simulink model "iap_device_boot_demo"  (Simulink 7.3)
settings: Solver=FixedStepDiscrete  SolverMode=SingleTasking  StartTime=0.0  StopTime=10.0  RelTol=1e-3
PreLoadFcn:
  | waijung.modelPreload; % Required for working with Waijung Blockset. Do not remove.
undefined symbols (not defined in the file): HSEOSC, Link, LQFP176, ST, STM32F417IG
libraries: simulink x22, stm32f4_flash_lib x12, stm32f4_canbus_lib x4, stm32f4_reset_lib x3, stm32f4_io_lib x3, stm32f4_boot_lib x2, stm32f4_crc_lib x2, stm32f4_device_config_lib x1
CloseFcn:
  | waijung.modelClose; % Required for working with Waijung Blockset. Do not remove.
settings Model: Creator=Krisada  LastModifiedBy=Krisada
settings OptimizationCC: OptimizeModelRefInitCode=on  LifeSpan=1
settings HardwareCC: ProdEndianess=LittleEndian  ProdHWDeviceType=ARM Compatible->Cortex - M4  TargetEndianess=LittleEndian  TargetHWDeviceType=ARM Compatible->Cortex - M4
settings RTWCC: SystemTargetFile=stm32f4.tlc  GenerateMakefile=off  TemplateMakefile=ert_default_tmf  Description=STM32F4 Target  ProcessScript=stm32f4_make_rtw_hook
settings CodeAppCC: IgnoreCustomStorageClasses=off
settings STFCustomTargetCC: ModelReferenceCompliant=off  CombineOutputUpdateFcns=on  ERTCustomFileBanners=on  SupportContinuousTime=off  SupportNonInlinedSFcns=off  SystemTargetFile=stm32f4.tlc
settings ERTTargetCC: MultiwordLength=2048  ModelReferenceCompliant=off  ParMdlRefBuildCompliant=off  CompOptLevelCompliant=off  ERTFirstTimeCompliant=off  ModelStepFunctionPrototypeControlCompliant=off  CPPClassGenCompliant=off  ExtModeMexFile=noextcomm  InlinedParameterPlacement=NonHierarchical  ERTSrcFileBannerTemplate=stm32f4_code_template.cgt  ERTHdrFileBannerTemplate=stm32f4_code_template.cgt  ERTDataSrcFileTemplate=stm32f4_code_template.cgt  ERTDataHdrFileTemplate=stm32f4_code_template.cgt  ERTCustomFileTemplate=stm32f4_file_process.tlc

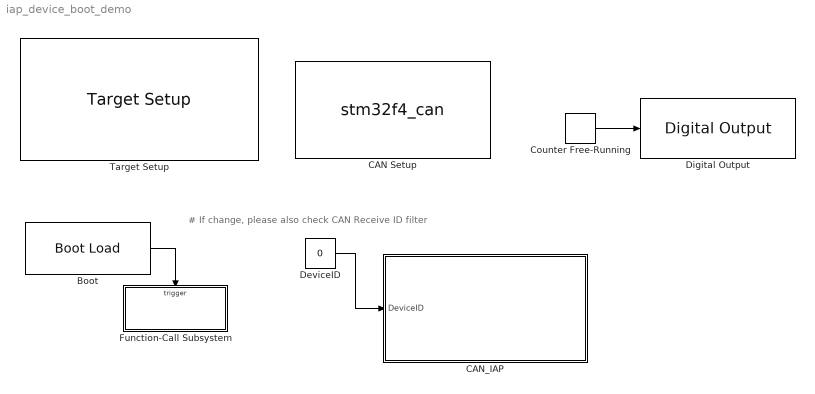
== system iap_device_boot_demo ==
  note: # If change,
      | please also check CAN Receive ID filter
  Boot : stm32f4_boot_lib/Boot Load  conf=Boot  flashorigin=0x8000000  flashlength=0x100000  enableisr=on  usersector=Sector 9: 0x080A0000 - 0x080BFFFF  sampletime=-1  sampletimestr=0.001  blockid=Boot  inputarray=[]  inputlabelarray={}  outputarray=[7]  outputlabelarray={'Call ISR'}  compat=0  confstr="[\"080A0000\",\"9\"]"
  CAN Setup : S-Function  FunctionName=stm32f4_can  Parameters=conf,canmodule,0,inputarray,outputarray,'','',confstr,sampletime,sampletimestr,blockid  EnableBusSupport=off  mask(stm32f4_can){conf=Setup, canmodule=1, advance=off, bitrate_select=125000, sjw=1tq, bs1=14tq, bs2=6tq, timingconf=Prescaler, brp=16, bitrate=125000, tq=3.8095e-007, remaptxpin=B9, remaprxpin=B8, sampletime=inf, sampletimestr=0.001, blockid=CANSetup, inputarray=[], inputlabelarray={}, outputarray=[], outputlabelarray={}, compat=0, confstr=["125000","16","B","9","B","8","1tq","14tq","6tq","ENABLE"], presc=16, txportstr=B, txpinstr=9, rxportstr=B, rxpinstr=8, lastmodule=1}
      mask prompts: conf "Configuration"; canmodule "CAN Module"; advance "Advance configuration"; bitrate_select "Baud rate (bps)"; sjw "Resync Jump Width (SJW)"; bs1 "Bit segment 1 (BS1) + PROP_SEG"; bs2 "Bit segment 2 (BS2)"; timingconf "Adjust"; brp "Baud rate prescaler (BRP)"; bitrate "Baud rate (bps)"; tq "Time Quantum (Second), tq"; remaptxpin "CAN Tx pin"; remaprxpin "CAN Rx pin"; sampletime "Sample time (sec)"; sampletimestr "Compiled sample time (sec) in string"; inputarray "Input port"; inputlabelarray "Input port label"; outputarray "Output port"; outputlabelarray "Output port label"; compat "Compatibility (Reserved for future use)"; confstr "Configuration String"; presc "Prescale"; txportstr "Tx port string"; txpinstr "Tx pin string"; rxportstr "Rx port string"; rxpinstr "Rx pin string"; lastmodule "Last module selected"
      mask help: This block setups CAN Module.
      mask init:
      | stm32f4_can_callback('init');
      mask Help: web(fullfile(waijungdocroot,'stm32f4_can_setup.htm'), '-browser')
      mask StyleString: popup(Setup),popup(1|2),checkbox,popup(125000|250000|500000|1000000),popup(1tq|2tq|3tq|4tq),popup(1tq|2tq|3tq|4tq|5tq|6tq|7tq|8tq|9tq|10tq|11tq|12tq|13tq|14tq|15tq|16tq),popup(1tq|2tq|3tq|4tq|5tq|6tq|7tq|8tq),popup(Prescaler|Baudrate),edit,edit,edit,popup(Not used|A12|B9|D1|H13),popup(Not used|A11|B8|D0|I9),edit,edit,edit,edit,edit,edit,edit,edit,edit,edit,edit,edit,edit,edit,edit
      mask CallbackString: |stm32f4_can_callback('canmodule');|stm32f4_can_callback('advance');|stm32f4_can_callback('bitrate_select');||stm32f4_can_callback('timingconf');|stm32f4_can_callback('timingconf');|stm32f4_can_callback('timingconf');|stm32f4_can_callback('timingconf');|stm32f4_can_callback('timingconf');||stm32f4_can_callback('remaptxpin');|stm32f4_can_callback('remaprxpin');|stm32f4_can_callback('sampletime');|stm32f4_can_callback('sampletimestr');|stm32f4_can_callback('blockid');||||||||||||
      mask Display: text(0.5, 0.5, 'CAN1_Setup\nSpeed (bps): 125000\nTx/Rx pin: B9/B8','ver','middle','hor','center');
  CAN_IAP : Subsystem  TreatAsAtomicUnit=on
  Counter Free-Running : simulink/Sources/Counter Free-Running  SystemSampleTime=-1  NumBits=16  tsamp=0.5
  DeviceID : Constant  Value=0  OutDataTypeMode=uint32  OutDataType=fixdt(1, 16)  OutScaling=2^0  OutDataTypeStr=uint32  SampleTime=0.001
  Digital Output : stm32f4_io_lib/Digital Output  use_bitband=on  port=D  speed=100  porttype=Push Pull  porttypestr=PP  use_pin0=off  use_pin1=off  use_pin2=off  use_pin3=off  use_pin4=off  use_pin5=off  use_pin6=off  use_pin7=off  use_pin8=off  use_pin9=off  use_pin10=off  use_pin11=off  use_pin12=off  use_pin13=off  use_pin14=off  use_pin15=on  pinstr=GPIO_Pin_15  usedpinarray="[0  0  0  0  0  0  0  0  0  0  0  0  0  0  0  1]"  bitbandingstr="#define DigitalOutput_D15 Peripheral_BB(GPIOD->ODR, 15)  /* Output pin */"  sampletime=-1  sampletimestr=0.5  blockid=DigitalOutput  enablecustomportlabel=off  globalinit=off  cinputportlabel=In1, In2  coutputportlabel=0
  Function-Call Subsystem : Subsystem  TreatAsAtomicUnit=on
  Target Setup : stm32f4_device_config_lib/Target Setup  Priority=100  compiler=GNU ARM  previous_compiler=GNU ARM  mcu=STM32F417IG (LQFP176)  mcustr=STM32F417IG  clockconfig=HSEOSC-8MHz  system_stm32f4xx_c_path=F:\trunk\targets\stm32f4_target\stm32f4\utils\system_stm32f4xx_default\STM32F40_41xxx\hseosc8mhz  showmemoryconfiguration=off  stacksize=0x2000  heapsize=0x2000  enableautocompiledownload=on  fullchiperase=on  programmerinterface=ST-Link  editctrlstr=on  compilercontrolstr=$(patsubst %, -I%, .) -mcpu=cortex-m4 -mthumb -mthumb-interwork -mfloat-abi=hard -mfpu=fpv4-sp-d16 -ffast-math -Wall -Wextra -Ofast  assemblercontrolstr=$(patsubst %, -I%, .) -mcpu=cortex-m4 -mthumb -mthumb-interwork -mfloat-abi=hard -mfpu=fpv4-sp-d16 -ffast-math -Wall -Wextra -Ofast -Wa,-amhls=$(<:.s=.lst) -D__STACK_SIZE=$(STACK_SIZE) -D__HEAP_SIZE=$(HEAP_SIZE)  linkercontrolstr=-T$(LD_SCRIPT) -g -Wl,-Map=$(MAP),--cref,--no-warn-mismatch -mcpu=cortex-m4 -mthumb -mthumb-interwork -mfloat-abi=hard -mfpu=fpv4-sp-d16 -specs=nosys.specs  runafterdownload=on  execprofile=None  profileruart=3  profilerbaud=500000  profilertxpin=D8  profilerinitstr=0.001,168000000,168000,500000,0  manualsetsampletime=off  sampletime=0.001  blockid=TargetSetup  systickreloadvalue=168000  hseval=8000000  lastprofileruart=3  hclk=168000000  flashorigin=0x8000000  flashlength=1024k  ramorigin=0x20000000  ramlength=128k  useextram=off
  wires:
  Boot/1 -> Function-Call Subsystem/Trigger
  DeviceID/1 -> CAN_IAP/1(DeviceID)
  Counter Free-Running/1 -> Digital Output/1

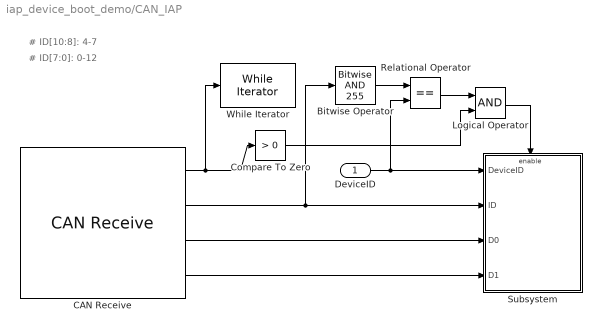
== system iap_device_boot_demo/CAN_IAP ==
  note: # ID[7:0]: 0-12
  note: # ID[10:8]: 4-7
  DeviceID : Inport  OutDataType=fixdt(1, 16)  OutScaling=2^0
  Bitwise Operator : simulink/Logic and Bit Operations/Bitwise Operator  logicop=AND  UseBitMask=on  BitMask=255  BitMaskRealWorld=Stored Integer
  CAN Receive : stm32f4_canbus_lib/CAN Receive  conf=Rx  canmodule=1  idtype=Standard  filtertype=Mask  id=hex2dec('400')  idmask=hex2dec('4F0')  enableisr=off  usedlc=off  datatype=uint32  data0type=uint32  data1type=uint32  data2type=Not used  data3type=Not used  data4type=Not used  data5type=Not used  data6type=Not used  data7type=Not used  buffersize=32  sampletime=-1  sampletimestr=-1  blockid=CAN_IAPCANReceive  inputarray=[]  inputlabelarray={}  outputarray=[ 5, 7, 7, 7]  outputlabelarray={ 'Msg Pending','ID', 'D0 (uint32)', 'D1 (uint32)' }  compat=0  confstr="[\"Standard\",\"Mask\",\"1024\",\"1264\",\"off\",\"uint32\",\"uint32\",\"Not used\",\"Not used\",\"Not used\",\"Not used\",\"Not used\",\"Not used\",\"32\",\"8000\",\"0\",\"9E00\",\"4\"]"
  Compare To Zero : simulink/Logic and Bit Operations/Compare To Zero  SystemSampleTime=-1  relop=>  LogicOutDataTypeMode=uint8  ZeroCross=off
  Logical Operator : Logic  AllPortsSameDT=off  OutDataTypeMode=boolean  LogicDataType=fixdt(0, 8)  OutDataTypeStr=boolean
  Relational Operator : RelationalOperator  Operator===  LogicOutDataTypeMode=boolean  LogicDataType=fixdt(0, 8)  OutDataTypeStr=boolean
  Subsystem : Subsystem
  While Iterator : WhileIterator  WhileBlockType=do-while
  wires:
  CAN Receive/1 -> Compare To Zero/1, While Iterator/1
  CAN Receive/4 -> Subsystem/4(D1)
  CAN Receive/2 -> Subsystem/2(ID), Bitwise Operator/1
  CAN Receive/3 -> Subsystem/3(D0)
  Relational Operator/1 -> Logical Operator/1
  Compare To Zero/1 -> Logical Operator/2
  Logical Operator/1 -> Subsystem/Enable
  Bitwise Operator/1 -> Relational Operator/1
  DeviceID/1 -> Subsystem/1(DeviceID), Relational Operator/2

== system iap_device_boot_demo/Function-Call Subsystem ==
  note: # 1. Stay in boot if PA0 pressed during Startup
  note: 2. Otherwise, check flash healthy
  function : TriggerPort  TriggerType=function-call
  Check Boot Pin : Subsystem  TreatAsAtomicUnit=on
  Check Flash : Subsystem
  Constant : Constant  OutDataType=fixdt(1, 16)  OutScaling=2^0
  wires:
  Constant/1 -> Check Boot Pin/Enable
  Check Boot Pin/1(Out1) -> Check Flash/Enable

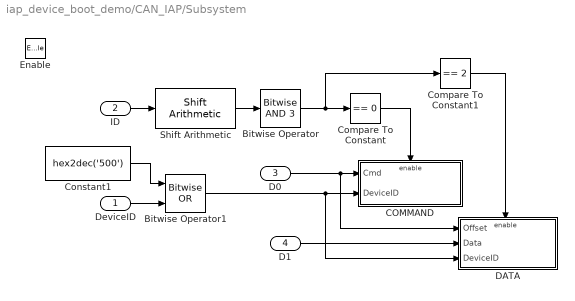
== system iap_device_boot_demo/CAN_IAP/Subsystem ==
  DeviceID : Inport
  ID : Inport  Port=2
  D0 : Inport  Port=3
  D1 : Inport  Port=4
  Enable : EnablePort
  Bitwise Operator : simulink/Logic and Bit Operations/Bitwise Operator  logicop=AND  UseBitMask=on  BitMask=3  BitMaskRealWorld=Stored Integer
  Bitwise Operator1 : simulink/Logic and Bit Operations/Bitwise Operator  logicop=OR  UseBitMask=off  NumInputPorts=2  BitMask=bin2dec('11011001')  BitMaskRealWorld=Stored Integer
  COMMAND : Subsystem  TreatAsAtomicUnit=on
  Compare To Constant : simulink/Logic and Bit Operations/Compare To Constant  SystemSampleTime=-1  relop===  const=0  LogicOutDataTypeMode=uint8  ZeroCross=off
  Compare To Constant1 : simulink/Logic and Bit Operations/Compare To Constant  SystemSampleTime=-1  relop===  const=2  LogicOutDataTypeMode=uint8  ZeroCross=off
  Constant1 : Constant  Value=hex2dec('500')  OutDataTypeMode=uint32  OutDataType=fixdt(1, 16)  OutScaling=2^0  OutDataTypeStr=uint32
  DATA : Subsystem  TreatAsAtomicUnit=on
  Shift Arithmetic : simulink/Logic and Bit Operations/Shift Arithmetic  SystemSampleTime=-1  nBitShiftRight=8  nBinPtShiftRight=0
  wires:
  Shift Arithmetic/1 -> Bitwise Operator/1
  Bitwise Operator/1 -> Compare To Constant1/1, Compare To Constant/1
  Compare To Constant/1 -> COMMAND/Enable
  D0/1 -> COMMAND/1(Cmd), DATA/1(Offset)
  Compare To Constant1/1 -> DATA/Enable
  ID/1 -> Shift Arithmetic/1
  D1/1 -> DATA/2(Data)
  Constant1/1 -> Bitwise Operator1/1
  DeviceID/1 -> Bitwise Operator1/2
  Bitwise Operator1/1 -> COMMAND/2(DeviceID), DATA/3(DeviceID)

== system iap_device_boot_demo/Function-Call Subsystem/Check Boot Pin ==
  Enable : EnablePort
  Digital Input : stm32f4_io_lib/Digital Input  port=A  speed=100  porttype=None  porttypestr=NOPULL  use_pin0=on  use_pin1=off  use_pin2=off  use_pin3=off  use_pin4=off  use_pin5=off  use_pin6=off  use_pin7=off  use_pin8=off  use_pin9=off  use_pin10=off  use_pin11=off  use_pin12=off  use_pin13=off  use_pin14=off  use_pin15=off  pinstr=GPIO_Pin_0  usedpinarray="[1  0  0  0  0  0  0  0  0  0  0  0  0  0  0  0]"  bitbandingstr="#define FunctionCallSubsystemCheckBootPinDigitalInput_A0 Peripheral_BB(GPIOA->IDR, 0)  /* Output pin */"  sampletime=inf  sampletimestr=-1  blockid=FunctionCallSubsystemCheckBootPinDigitalInput  enablecustomportlabel=off  glabalinit=off  cinputportlabel=In1, In2  coutputportlabel=Out1, Out2
  Logical Operator : Logic  Operator=NOT  AllPortsSameDT=off  OutDataTypeMode=boolean  LogicDataType=fixdt(0, 8)  OutDataTypeStr=boolean
  Out1 : Outport  OutDataType=fixdt(1, 16)  OutScaling=2^0
  wires:
  Digital Input/1 -> Logical Operator/1
  Logical Operator/1 -> Out1/1

== system iap_device_boot_demo/Function-Call Subsystem/Check Flash ==
  note: #  Check if firmwar has valid stack address,
      | reduce proces to check CRC32 when firmware invalid
  note: ### Sector C location: Sector_6
  Enable : EnablePort
  Check Sector B : Subsystem  TreatAsAtomicUnit=on
  Check Sector C : Subsystem
  Logical Operator : Logic  Operator=NOT  AllPortsSameDT=off  OutDataTypeMode=boolean  LogicDataType=fixdt(0, 8)  OutDataTypeStr=boolean
  Upgrade Firmware : Subsystem  TreatAsAtomicUnit=on
  wires:
  Check Sector C/1(Sector Valid) -> Upgrade Firmware/Enable, Logical Operator/1
  Logical Operator/1 -> Check Sector B/Enable

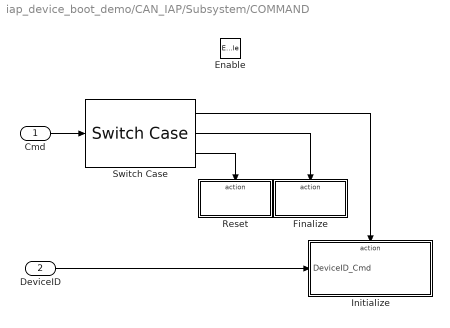
== system iap_device_boot_demo/CAN_IAP/Subsystem/COMMAND ==
  Cmd : Inport  OutDataType=fixdt(1, 16)  OutScaling=2^0
  DeviceID : Inport  Port=2  OutDataType=fixdt(1, 16)  OutScaling=2^0
  Enable : EnablePort
  Finalize : Subsystem  TreatAsAtomicUnit=on
  Initialize : Subsystem  TreatAsAtomicUnit=on
  Reset : Subsystem  TreatAsAtomicUnit=on
  Switch Case : SwitchCase  CaseConditions={0,1,2}  CaseShowDefault=off
  wires:
  Cmd/1 -> Switch Case/1
  Switch Case/1 -> Initialize/Action
  Switch Case/2 -> Finalize/Action
  Switch Case/3 -> Reset/Action
  DeviceID/1 -> Initialize/1(DeviceID_Cmd)

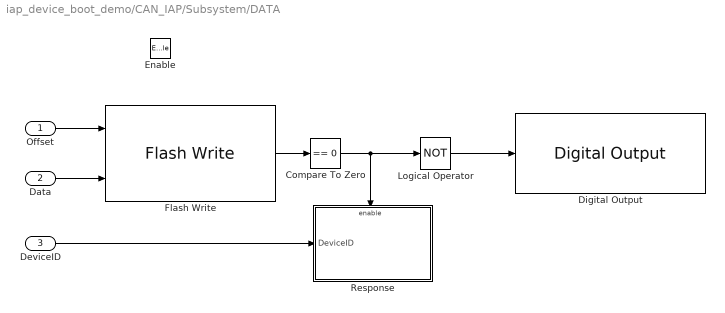
== system iap_device_boot_demo/CAN_IAP/Subsystem/DATA ==
  Offset : Inport  OutDataType=fixdt(1, 16)  OutScaling=2^0
  Data : Inport  Port=2  OutDataType=fixdt(1, 16)  OutScaling=2^0
  DeviceID : Inport  Port=3  OutDataType=fixdt(1, 16)  OutScaling=2^0
  Enable : EnablePort
  Compare To Zero : simulink/Logic and Bit Operations/Compare To Zero  SystemSampleTime=-1  relop===  LogicOutDataTypeMode=uint8  ZeroCross=off
  Digital Output : stm32f4_io_lib/Digital Output  use_bitband=on  port=D  speed=100  porttype=Push Pull  porttypestr=PP  use_pin0=off  use_pin1=off  use_pin2=off  use_pin3=off  use_pin4=off  use_pin5=off  use_pin6=off  use_pin7=off  use_pin8=off  use_pin9=off  use_pin10=off  use_pin11=off  use_pin12=off  use_pin13=off  use_pin14=on  use_pin15=off  pinstr=GPIO_Pin_14  usedpinarray="[0  0  0  0  0  0  0  0  0  0  0  0  0  0  1  0]"  bitbandingstr="#define CAN_IAPSubsystemDATADigitalOutput_D14 Peripheral_BB(GPIOD->ODR, 14)  /* Output pin */"  sampletime=-1  sampletimestr=-1  blockid=CAN_IAPSubsystemDATADigitalOutput  enablecustomportlabel=off  globalinit=off  cinputportlabel=In1, In2  coutputportlabel=0
  Flash Write : stm32f4_flash_lib/Flash Write  conf=Program  transfer=Blocking  flashsector=Sector 6: 0x08040000 - 0x0805FFFF  datatype=uint32  datacount=1  enablestatus=on  sampletime=-1  sampletimestr=-1  blockid=CAN_IAPSubsystemDATAFlashWrite  inputarray=[-1,7]  inputlabelarray={'Offset ', 'Data (uint32)'}  outputarray=[3]  outputlabelarray={'Status'}  compat=0  confstr="[\"Blocking\",\"uint32\",\"on\",\"20000\",\"08040000\",\"6\"]"
  Logical Operator : Logic  Operator=NOT  AllPortsSameDT=off  OutDataTypeMode=boolean  LogicDataType=fixdt(0, 8)  OutDataTypeStr=boolean
  Response : Subsystem
  wires:
  Offset/1 -> Flash Write/1
  Data/1 -> Flash Write/2
  Compare To Zero/1 -> Response/Enable, Logical Operator/1
  Flash Write/1 -> Compare To Zero/1
  DeviceID/1 -> Response/1(DeviceID)
  Logical Operator/1 -> Digital Output/1

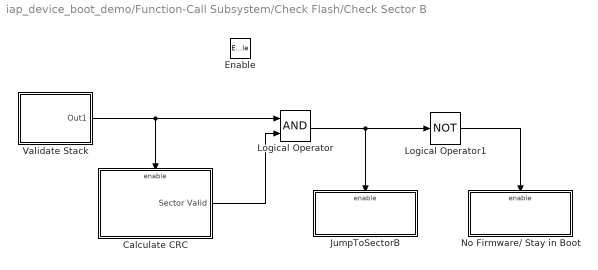
== system iap_device_boot_demo/Function-Call Subsystem/Check Flash/Check Sector B ==
  Enable : EnablePort
  Calculate CRC : Subsystem  TreatAsAtomicUnit=on
  JumpToSectorB : Subsystem  TreatAsAtomicUnit=on
  Logical Operator : Logic  AllPortsSameDT=off  OutDataTypeMode=boolean  LogicDataType=fixdt(0, 8)  OutDataTypeStr=boolean
  Logical Operator1 : Logic  Operator=NOT  AllPortsSameDT=off  OutDataTypeMode=boolean  LogicDataType=fixdt(0, 8)  OutDataTypeStr=boolean
  No Firmware/ Stay in Boot : Subsystem  TreatAsAtomicUnit=on
  Validate Stack : Subsystem
  wires:
  Validate Stack/1(Out1) -> Calculate CRC/Enable, Logical Operator/1
  Calculate CRC/1(Sector Valid) -> Logical Operator/2
  Logical Operator/1 -> JumpToSectorB/Enable, Logical Operator1/1
  Logical Operator1/1 -> No Firmware/ Stay in Boot/Enable

== system iap_device_boot_demo/Function-Call Subsystem/Check Flash/Check Sector C ==
  Calculate CRC : Subsystem  TreatAsAtomicUnit=on
  Logical Operator : Logic  AllPortsSameDT=off  OutDataTypeMode=boolean  LogicDataType=fixdt(0, 8)  OutDataTypeStr=boolean
  Validate Stack : Subsystem
  Sector Valid : Outport  OutDataType=fixdt(1, 16)  OutScaling=2^0
  wires:
  Validate Stack/1(Out1) -> Calculate CRC/Enable, Logical Operator/1
  Calculate CRC/1(Sector Valid) -> Logical Operator/2
  Logical Operator/1 -> Sector Valid/1

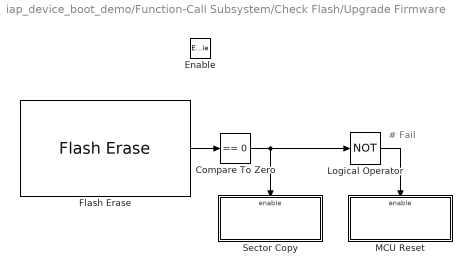
== system iap_device_boot_demo/Function-Call Subsystem/Check Flash/Upgrade Firmware ==
  note: # Fail
  Enable : EnablePort
  Compare To Zero : simulink/Logic and Bit Operations/Compare To Zero  SystemSampleTime=-1  relop===  LogicOutDataTypeMode=uint8  ZeroCross=off
  Flash Erase : stm32f4_flash_lib/Flash Erase  conf=Erase  transfer=Blocking  flashsector=Sector 5: 0x08020000 - 0x0803FFFF  datatype=uint32  datacount=1  enablestatus=on  sampletime=-1  sampletimestr=-1  blockid=FunctionCallSubsystemCheckFlashUpgradeFirmwareFlashErase  inputarray=[]  inputlabelarray={}  outputarray=[3]  outputlabelarray={'Status'}  compat=0  confstr="[\"Blocking\",\"on\",\"08020000\",\"5\"]"
  Logical Operator : Logic  Operator=NOT  AllPortsSameDT=off  OutDataTypeMode=boolean  LogicDataType=fixdt(0, 8)  OutDataTypeStr=boolean
  MCU Reset : Subsystem  TreatAsAtomicUnit=on
  Sector Copy : Subsystem  TreatAsAtomicUnit=on
  wires:
  Flash Erase/1 -> Compare To Zero/1
  Compare To Zero/1 -> Sector Copy/Enable, Logical Operator/1
  Logical Operator/1 -> MCU Reset/Enable

== system iap_device_boot_demo/CAN_IAP/Subsystem/COMMAND/Finalize ==
  Action Port : ActionPort  ActionType=case

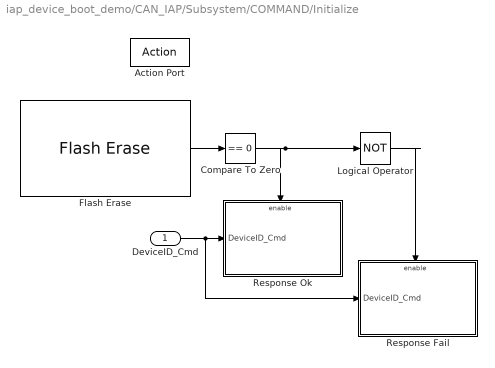
== system iap_device_boot_demo/CAN_IAP/Subsystem/COMMAND/Initialize ==
  DeviceID_Cmd : Inport  OutDataType=fixdt(1, 16)  OutScaling=2^0
  Action Port : ActionPort  ActionType=case
  Compare To Zero : simulink/Logic and Bit Operations/Compare To Zero  SystemSampleTime=-1  relop===  LogicOutDataTypeMode=uint8  ZeroCross=off
  Flash Erase : stm32f4_flash_lib/Flash Erase  conf=Erase  transfer=Blocking  flashsector=Sector 6: 0x08040000 - 0x0805FFFF  datatype=uint32  datacount=1  enablestatus=on  sampletime=-1  sampletimestr=-1  blockid=CAN_IAPSubsystemCOMMANDInitializeFlashErase  inputarray=[]  inputlabelarray={}  outputarray=[3]  outputlabelarray={'Status'}  compat=0  confstr="[\"Blocking\",\"on\",\"08040000\",\"6\"]"
  Logical Operator : Logic  Operator=NOT  AllPortsSameDT=off  OutDataTypeMode=boolean  LogicDataType=fixdt(0, 8)  OutDataTypeStr=boolean
  Response Fail : Subsystem
  Response Ok : Subsystem
  wires:
  Flash Erase/1 -> Compare To Zero/1
  Compare To Zero/1 -> Response Ok/Enable, Logical Operator/1
  Logical Operator/1 -> Response Fail/Enable
  DeviceID_Cmd/1 -> Response Ok/1(DeviceID_Cmd), Response Fail/1(DeviceID_Cmd)

== system iap_device_boot_demo/CAN_IAP/Subsystem/COMMAND/Reset ==
  Action Port : ActionPort  ActionType=case
  System Reset : stm32f4_reset_lib/System Reset  conf=<empty>  sampletime=inf  sampletimestr=-1  blockid=CAN_IAPSubsystemCOMMANDResetSystemReset  inputarray=[]  inputlabelarray={}  outputarray=[]  outputlabelarray={}  compat=0  confstr="[\"Param1\",\"Param1\"]"

== system iap_device_boot_demo/CAN_IAP/Subsystem/DATA/Response ==
  DeviceID : Inport  OutDataType=fixdt(1, 16)  OutScaling=2^0
  Enable : EnablePort
  CAN Transmit : stm32f4_canbus_lib/CAN Transmit  conf=Tx  canmodule=1  transfer=Blocking  timeout=0.001  idtype=Standard  specificid=off  id=hex2dec('400')  specificdlc=on  dlc=8  enablestatus=off  datatype=uint32  data0type=uint32  data1type=uint32  data2type=Not used  data3type=Not used  data4type=Not used  data5type=Not used  data6type=Not used  data7type=Not used  inputarray=[ -1, 7, 7]  inputlabelarray={ 'ID', 'D0 (uint32)', 'D1 (uint32)' }  outputarray=[]  outputlabelarray={}  sampletime=-1  sampletimestr=-1  blockid=CAN_IAPSubsystemDATAResponseCANTransmit  compat=0  confstr="[\"Blocking\",\"0.001\",\"Standard\",\"off\",\"1024\",\"on\",\"8\",\"off\",\"uint32\",\"uint32\",\"Not used\",\"Not used\",\"Not used\",\"Not used\",\"Not used\",\"Not used\"]"
  Constant : Constant  Value=0  OutDataTypeMode=uint32  OutDataType=fixdt(1, 16)  OutScaling=2^0  OutDataTypeStr=uint32
  wires:
  DeviceID/1 -> CAN Transmit/1
  Constant/1 -> CAN Transmit/3, CAN Transmit/2

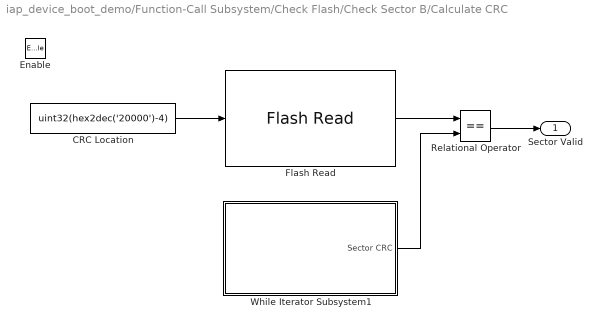
== system iap_device_boot_demo/Function-Call Subsystem/Check Flash/Check Sector B/Calculate CRC ==
  Enable : EnablePort
  CRC Location : Constant  Value=uint32(hex2dec('20000')-4)  OutDataType=fixdt(1, 16)  OutScaling=2^0
  Flash Read : stm32f4_flash_lib/Flash Read  conf=Read  transfer=Blocking  flashsector=Sector 5: 0x08020000 - 0x0803FFFF  datatype=uint32  datacount=1  enablestatus=off  sampletime=-1  sampletimestr=-1  blockid=FunctionCallSubsystemCheckFlashCheckSectorBCalculateCRCFlashRead  inputarray=[-1]  inputlabelarray={'Offset '}  outputarray=[7]  outputlabelarray={'Data (uint32)'}  compat=0  confstr="[\"uint32\",\"20000\",\"08020000\",\"5\",\"off\"]"
  Relational Operator : RelationalOperator  Operator===  LogicOutDataTypeMode=boolean  LogicDataType=fixdt(0, 8)  OutDataTypeStr=boolean
  While Iterator Subsystem1 : Subsystem  TreatAsAtomicUnit=on
  Sector Valid : Outport  OutDataType=fixdt(1, 16)  OutScaling=2^0
  wires:
  CRC Location/1 -> Flash Read/1
  While Iterator Subsystem1/1(Sector CRC) -> Relational Operator/2
  Flash Read/1 -> Relational Operator/1
  Relational Operator/1 -> Sector Valid/1

== system iap_device_boot_demo/Function-Call Subsystem/Check Flash/Check Sector B/JumpToSectorB ==
  Enable : EnablePort
  Boot : stm32f4_boot_lib/Jump Sector  conf=Goto  flashorigin=0x8000000  flashlength=0x100000  enableisr=off  usersector=Sector 5: 0x08020000 - 0x0803FFFF  sampletime=inf  sampletimestr=-1  blockid=FunctionCallSubsystemCheckFlashCheckSectorBJumpToSectorBBoot  inputarray=[]  inputlabelarray={}  outputarray=[]  outputlabelarray={}  compat=0  confstr="[\"08020000\",\"5\"]"

== system iap_device_boot_demo/Function-Call Subsystem/Check Flash/Check Sector B/No Firmware/ Stay in Boot ==
  Enable : EnablePort

== system iap_device_boot_demo/Function-Call Subsystem/Check Flash/Check Sector B/Validate Stack ==
  Bitwise Operator : simulink/Logic and Bit Operations/Bitwise Operator  logicop=AND  UseBitMask=on  BitMask=hex2dec('2FFE0000')  BitMaskRealWorld=Stored Integer
  Compare To 0x20000000 : simulink/Logic and Bit Operations/Compare To Constant  SystemSampleTime=-1  relop===  const=hex2dec('20000000')  LogicOutDataTypeMode=boolean  ZeroCross=off
  Read Stack1 : stm32f4_flash_lib/Flash Read  conf=Read  transfer=Blocking  flashsector=Sector 5: 0x08020000 - 0x0803FFFF  datatype=uint32  datacount=1  enablestatus=off  sampletime=-1  sampletimestr=-1  blockid=FunctionCallSubsystemCheckFlashCheckSectorBValidateStackReadStack1  inputarray=[-1]  inputlabelarray={'Offset '}  outputarray=[7]  outputlabelarray={'Data (uint32)'}  compat=0  confstr="[\"uint32\",\"20000\",\"08020000\",\"5\",\"off\"]"
  Stack Location : Constant  Value=0  OutDataType=fixdt(1, 16)  OutScaling=2^0
  Out1 : Outport
  wires:
  Read Stack1/1 -> Bitwise Operator/1
  Stack Location/1 -> Read Stack1/1
  Bitwise Operator/1 -> Compare To 0x20000000/1
  Compare To 0x20000000/1 -> Out1/1

== system iap_device_boot_demo/Function-Call Subsystem/Check Flash/Check Sector C/Calculate CRC ==
  Enable : EnablePort
  CRC Location : Constant  Value=uint32(hex2dec('20000')-4)  OutDataType=fixdt(1, 16)  OutScaling=2^0
  Flash Read : stm32f4_flash_lib/Flash Read  conf=Read  transfer=Blocking  flashsector=Sector 6: 0x08040000 - 0x0805FFFF  datatype=uint32  datacount=1  enablestatus=off  sampletime=-1  sampletimestr=-1  blockid=FunctionCallSubsystemCheckFlashCheckSectorCCalculateCRCFlashRead  inputarray=[-1]  inputlabelarray={'Offset '}  outputarray=[7]  outputlabelarray={'Data (uint32)'}  compat=0  confstr="[\"uint32\",\"20000\",\"08040000\",\"6\",\"off\"]"
  Relational Operator : RelationalOperator  Operator===  LogicOutDataTypeMode=boolean  LogicDataType=fixdt(0, 8)  OutDataTypeStr=boolean
  While Iterator Subsystem : Subsystem  TreatAsAtomicUnit=on
  Sector Valid : Outport  OutDataType=fixdt(1, 16)  OutScaling=2^0
  wires:
  CRC Location/1 -> Flash Read/1
  While Iterator Subsystem/1(Sector CRC) -> Relational Operator/2
  Flash Read/1 -> Relational Operator/1
  Relational Operator/1 -> Sector Valid/1

== system iap_device_boot_demo/Function-Call Subsystem/Check Flash/Check Sector C/Validate Stack ==
  Bitwise Operator : simulink/Logic and Bit Operations/Bitwise Operator  logicop=AND  UseBitMask=on  BitMask=hex2dec('2FFE0000')  BitMaskRealWorld=Stored Integer
  Compare To 0x20000000 : simulink/Logic and Bit Operations/Compare To Constant  SystemSampleTime=-1  relop===  const=hex2dec('20000000')  LogicOutDataTypeMode=boolean  ZeroCross=off
  Read Stack1 : stm32f4_flash_lib/Flash Read  conf=Read  transfer=Blocking  flashsector=Sector 6: 0x08040000 - 0x0805FFFF  datatype=uint32  datacount=1  enablestatus=off  sampletime=-1  sampletimestr=-1  blockid=FunctionCallSubsystemCheckFlashCheckSectorCValidateStackReadStack1  inputarray=[-1]  inputlabelarray={'Offset '}  outputarray=[7]  outputlabelarray={'Data (uint32)'}  compat=0  confstr="[\"uint32\",\"20000\",\"08040000\",\"6\",\"off\"]"
  Stack Location : Constant  Value=0  OutDataType=fixdt(1, 16)  OutScaling=2^0
  Out1 : Outport
  wires:
  Read Stack1/1 -> Bitwise Operator/1
  Stack Location/1 -> Read Stack1/1
  Bitwise Operator/1 -> Compare To 0x20000000/1
  Compare To 0x20000000/1 -> Out1/1

== system iap_device_boot_demo/Function-Call Subsystem/Check Flash/Upgrade Firmware/MCU Reset ==
  Enable : EnablePort
  System Reset : stm32f4_reset_lib/System Reset  conf=<empty>  sampletime=inf  sampletimestr=-1  blockid=FunctionCallSubsystemCheckFlashUpgradeFirmwareMCUResetSystemReset  inputarray=[]  inputlabelarray={}  outputarray=[]  outputlabelarray={}  compat=0  confstr="[\"Param1\",\"Param1\"]"

== system iap_device_boot_demo/Function-Call Subsystem/Check Flash/Upgrade Firmware/Sector Copy ==
  Enable : EnablePort
  Clone Sector : Subsystem  TreatAsAtomicUnit=on
  Finallize : Subsystem  TreatAsAtomicUnit=on
  wires:
  Clone Sector/1(Success) -> Finallize/Enable

== system iap_device_boot_demo/CAN_IAP/Subsystem/COMMAND/Initialize/Response Fail ==
  DeviceID_Cmd : Inport  OutDataType=fixdt(1, 16)  OutScaling=2^0
  Enable : EnablePort
  CAN Transmit : stm32f4_canbus_lib/CAN Transmit  conf=Tx  canmodule=1  transfer=Blocking  timeout=0.001  idtype=Standard  specificid=off  id=hex2dec('400')  specificdlc=on  dlc=8  enablestatus=off  datatype=uint32  data0type=uint32  data1type=uint32  data2type=Not used  data3type=Not used  data4type=Not used  data5type=Not used  data6type=Not used  data7type=Not used  inputarray=[ -1, 7, 7]  inputlabelarray={ 'ID', 'D0 (uint32)', 'D1 (uint32)' }  outputarray=[]  outputlabelarray={}  sampletime=-1  sampletimestr=-1  blockid=CAN_IAPSubsystemCOMMANDInitializeResponseFailCANTransmit  compat=0  confstr="[\"Blocking\",\"0.001\",\"Standard\",\"off\",\"1024\",\"on\",\"8\",\"off\",\"uint32\",\"uint32\",\"Not used\",\"Not used\",\"Not used\",\"Not used\",\"Not used\",\"Not used\"]"
  Constant : Constant  Value=0  OutDataTypeMode=uint32  OutDataType=fixdt(1, 16)  OutScaling=2^0  OutDataTypeStr=uint32
  Constant1 : Constant  OutDataTypeMode=uint32  OutDataType=fixdt(1, 16)  OutScaling=2^0  OutDataTypeStr=uint32
  wires:
  Constant/1 -> CAN Transmit/3
  Constant1/1 -> CAN Transmit/2
  DeviceID_Cmd/1 -> CAN Transmit/1

== system iap_device_boot_demo/CAN_IAP/Subsystem/COMMAND/Initialize/Response Ok ==
  DeviceID_Cmd : Inport  OutDataType=fixdt(1, 16)  OutScaling=2^0
  Enable : EnablePort
  CAN Transmit : stm32f4_canbus_lib/CAN Transmit  conf=Tx  canmodule=1  transfer=Blocking  timeout=0.001  idtype=Standard  specificid=off  id=hex2dec('400')  specificdlc=on  dlc=8  enablestatus=off  datatype=uint32  data0type=uint32  data1type=uint32  data2type=Not used  data3type=Not used  data4type=Not used  data5type=Not used  data6type=Not used  data7type=Not used  inputarray=[ -1, 7, 7]  inputlabelarray={ 'ID', 'D0 (uint32)', 'D1 (uint32)' }  outputarray=[]  outputlabelarray={}  sampletime=-1  sampletimestr=-1  blockid=CAN_IAPSubsystemCOMMANDInitializeResponseOkCANTransmit  compat=0  confstr="[\"Blocking\",\"0.001\",\"Standard\",\"off\",\"1024\",\"on\",\"8\",\"off\",\"uint32\",\"uint32\",\"Not used\",\"Not used\",\"Not used\",\"Not used\",\"Not used\",\"Not used\"]"
  Constant : Constant  Value=0  OutDataTypeMode=uint32  OutDataType=fixdt(1, 16)  OutScaling=2^0  OutDataTypeStr=uint32
  wires:
  Constant/1 -> CAN Transmit/3, CAN Transmit/2
  DeviceID_Cmd/1 -> CAN Transmit/1

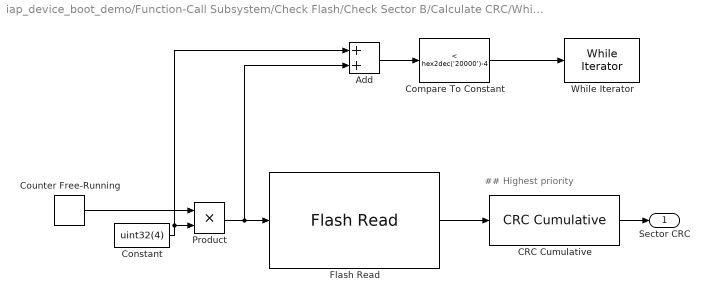
== system iap_device_boot_demo/Function-Call Subsystem/Check Flash/Check Sector B/Calculate CRC/While Iterator Subsystem1 ==
  note: ## Highest priority
  Add : Sum  OutDataType=fixdt(1, 16)  OutScaling=2^-10
  CRC Cumulative : stm32f4_crc_lib/CRC Cumulative  Priority=0  conf=Cumulative  sampletime=-1  sampletimestr=-1  blockid=FunctionCallSubsystemCheckFlashCheckSectorBCalculateCRCWhileIteratorSubsystem1CRCCumulative  inputarray=[7]  inputlabelarray={'uint32'}  outputarray=[7]  outputlabelarray={'uint32'}  compat=0  confstr="[\"Param1\",\"Param1\"]"
  Compare To Constant : simulink/Logic and Bit Operations/Compare To Constant  SystemSampleTime=-1  relop=<  const=hex2dec('20000')-4  LogicOutDataTypeMode=uint8  ZeroCross=off
  Constant : Constant  Value=uint32(4)  OutDataType=fixdt(1, 16)  OutScaling=2^0
  Counter Free-Running : simulink/Sources/Counter Free-Running  SystemSampleTime=-1  NumBits=32  tsamp=-1
  Flash Read : stm32f4_flash_lib/Flash Read  conf=Read  transfer=Blocking  flashsector=Sector 5: 0x08020000 - 0x0803FFFF  datatype=uint32  datacount=1  enablestatus=on  sampletime=-1  sampletimestr=-1  blockid=FunctionCallSubsystemCheckFlashCheckSectorBCalculateCRCWhileIteratorSubsystem1FlashRead  inputarray=[-1]  inputlabelarray={'Offset '}  outputarray=[7]  outputlabelarray={'Data (uint32)'}  compat=0  confstr="[\"uint32\",\"20000\",\"08020000\",\"5\",\"on\"]"
  Product : Product  OutDataTypeMode=uint32  OutDataType=fixdt(1, 16)  OutScaling=2^0  OutDataTypeStr=uint32  RndMeth=Zero
  While Iterator : WhileIterator  Priority=1  MaxIters=-1  WhileBlockType=do-while
  Sector CRC : Outport  OutDataType=fixdt(1, 16)  OutScaling=2^0
  wires:
  Add/1 -> Compare To Constant/1
  CRC Cumulative/1 -> Sector CRC/1
  Flash Read/1 -> CRC Cumulative/1
  Constant/1 -> Add/1, Product/2
  Product/1 -> Add/2, Flash Read/1
  Compare To Constant/1 -> While Iterator/1
  Counter Free-Running/1 -> Product/1

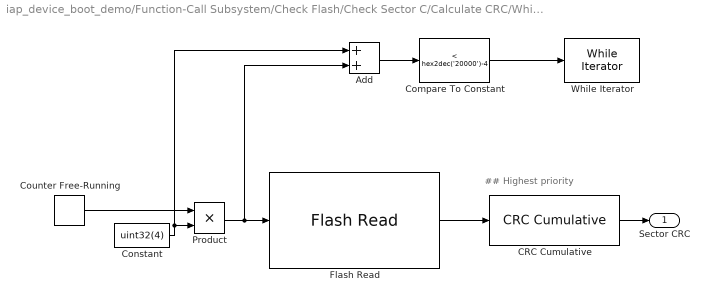
== system iap_device_boot_demo/Function-Call Subsystem/Check Flash/Check Sector C/Calculate CRC/While Iterator Subsystem ==
  note: ## Highest priority
  Add : Sum  OutDataType=fixdt(1, 16)  OutScaling=2^-10
  CRC Cumulative : stm32f4_crc_lib/CRC Cumulative  Priority=0  conf=Cumulative  sampletime=-1  sampletimestr=-1  blockid=FunctionCallSubsystemCheckFlashCheckSectorCCalculateCRCWhileIteratorSubsystemCRCCumulative  inputarray=[7]  inputlabelarray={'uint32'}  outputarray=[7]  outputlabelarray={'uint32'}  compat=0  confstr="[\"Param1\",\"Param1\"]"
  Compare To Constant : simulink/Logic and Bit Operations/Compare To Constant  SystemSampleTime=-1  relop=<  const=hex2dec('20000')-4  LogicOutDataTypeMode=uint8  ZeroCross=off
  Constant : Constant  Value=uint32(4)  OutDataType=fixdt(1, 16)  OutScaling=2^0
  Counter Free-Running : simulink/Sources/Counter Free-Running  SystemSampleTime=-1  NumBits=32  tsamp=-1
  Flash Read : stm32f4_flash_lib/Flash Read  conf=Read  transfer=Blocking  flashsector=Sector 6: 0x08040000 - 0x0805FFFF  datatype=uint32  datacount=1  enablestatus=on  sampletime=-1  sampletimestr=-1  blockid=FunctionCallSubsystemCheckFlashCheckSectorCCalculateCRCWhileIteratorSubsystemFlashRead  inputarray=[-1]  inputlabelarray={'Offset '}  outputarray=[7]  outputlabelarray={'Data (uint32)'}  compat=0  confstr="[\"uint32\",\"20000\",\"08040000\",\"6\",\"on\"]"
  Product : Product  OutDataTypeMode=uint32  OutDataType=fixdt(1, 16)  OutScaling=2^0  OutDataTypeStr=uint32  RndMeth=Zero
  While Iterator : WhileIterator  Priority=1  MaxIters=-1  WhileBlockType=do-while
  Sector CRC : Outport  OutDataType=fixdt(1, 16)  OutScaling=2^0
  wires:
  Counter Free-Running/1 -> Product/1
  Compare To Constant/1 -> While Iterator/1
  Product/1 -> Flash Read/1, Add/2
  Constant/1 -> Product/2, Add/1
  Flash Read/1 -> CRC Cumulative/1
  CRC Cumulative/1 -> Sector CRC/1
  Add/1 -> Compare To Constant/1

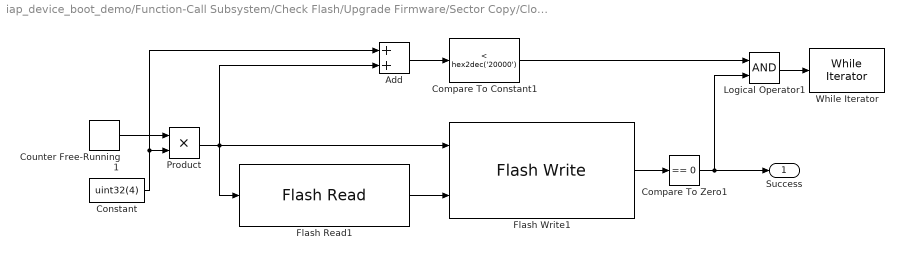
== system iap_device_boot_demo/Function-Call Subsystem/Check Flash/Upgrade Firmware/Sector Copy/Clone Sector ==
  Add : Sum  OutDataType=fixdt(1, 16)  OutScaling=2^-10
  Compare To Constant1 : simulink/Logic and Bit Operations/Compare To Constant  SystemSampleTime=-1  relop=<  const=hex2dec('20000')  LogicOutDataTypeMode=uint8  ZeroCross=off
  Compare To Zero1 : simulink/Logic and Bit Operations/Compare To Zero  SystemSampleTime=-1  relop===  LogicOutDataTypeMode=uint8  ZeroCross=off
  Constant : Constant  Value=uint32(4)  OutDataType=fixdt(1, 16)  OutScaling=2^0
  Counter Free-Running1 : simulink/Sources/Counter Free-Running  SystemSampleTime=-1  NumBits=32  tsamp=-1
  Flash Read1 : stm32f4_flash_lib/Flash Read  conf=Read  transfer=Blocking  flashsector=Sector 6: 0x08040000 - 0x0805FFFF  datatype=uint32  datacount=1  enablestatus=on  sampletime=-1  sampletimestr=-1  blockid=FunctionCallSubsystemCheckFlashUpgradeFirmwareSectorCopyCloneSectorFlashRead1  inputarray=[-1]  inputlabelarray={'Offset '}  outputarray=[7]  outputlabelarray={'Data (uint32)'}  compat=0  confstr="[\"uint32\",\"20000\",\"08040000\",\"6\",\"on\"]"
  Flash Write1 : stm32f4_flash_lib/Flash Write  conf=Program  transfer=Blocking  flashsector=Sector 5: 0x08020000 - 0x0803FFFF  datatype=uint32  datacount=1  enablestatus=on  sampletime=-1  sampletimestr=-1  blockid=FunctionCallSubsystemCheckFlashUpgradeFirmwareSectorCopyCloneSectorFlashWrite1  inputarray=[-1,7]  inputlabelarray={'Offset ', 'Data (uint32)'}  outputarray=[3]  outputlabelarray={'Status'}  compat=0  confstr="[\"Blocking\",\"uint32\",\"on\",\"20000\",\"08020000\",\"5\"]"
  Logical Operator1 : Logic  AllPortsSameDT=off  OutDataTypeMode=boolean  LogicDataType=fixdt(0, 8)  OutDataTypeStr=boolean
  Product : Product  OutDataTypeMode=uint32  OutDataType=fixdt(1, 16)  OutScaling=2^0  OutDataTypeStr=uint32  RndMeth=Zero
  While Iterator : WhileIterator  MaxIters=-1  WhileBlockType=do-while
  Success : Outport  OutDataType=fixdt(1, 16)  OutScaling=2^0
  wires:
  Counter Free-Running1/1 -> Product/1
  Product/1 -> Flash Read1/1, Add/2, Flash Write1/1
  Constant/1 -> Product/2, Add/1
  Flash Read1/1 -> Flash Write1/2
  Add/1 -> Compare To Constant1/1
  Flash Write1/1 -> Compare To Zero1/1
  Compare To Constant1/1 -> Logical Operator1/1
  Logical Operator1/1 -> While Iterator/1
  Compare To Zero1/1 -> Success/1, Logical Operator1/2

== system iap_device_boot_demo/Function-Call Subsystem/Check Flash/Upgrade Firmware/Sector Copy/Finallize ==
  note: ## Erase block higher priority
  Enable : EnablePort
  Erase Sector C : stm32f4_flash_lib/Flash Erase  Priority=1  conf=Erase  transfer=Blocking  flashsector=Sector 6: 0x08040000 - 0x0805FFFF  datatype=uint32  datacount=1  enablestatus=off  sampletime=-1  sampletimestr=-1  blockid=FunctionCallSubsystemCheckFlashUpgradeFirmwareSectorCopyFinallizeEraseSectorC  inputarray=[]  inputlabelarray={}  outputarray=[]  outputlabelarray={}  compat=0  confstr="[\"Blocking\",\"off\",\"08040000\",\"6\"]"
  System Reset : stm32f4_reset_lib/System Reset  Priority=2  conf=<empty>  sampletime=inf  sampletimestr=-1  blockid=FunctionCallSubsystemCheckFlashUpgradeFirmwareSectorCopyFinallizeSystemReset  inputarray=[]  inputlabelarray={}  outputarray=[]  outputlabelarray={}  compat=0  confstr="[\"Param1\",\"Param1\"]"
